simulink model "mex_block"  (Simulink 7.9)
settings: Solver=ode45  StartTime=0.0  StopTime=10.0  RelTol=1e-3
settings Model: Creator=adam  LastModifiedBy=adam

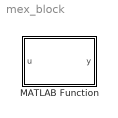
== system mex_block ==
  MATLAB Function : MATLAB Function  TreatAsAtomicUnit=on

== matlab function MATLAB Function ==
  data: u input double; y output double
function y = fcn(u)
 
%#codegen
mex *.cpp
